simulink model "SimulinkTesting"  (R2019a)
settings: Solver=VariableStepAuto  StartTime=0.0  StopTime=1  MaxStep=0.2  MinStep=0.1  RelTol=1e-3
settings Model: Creator=Devin  LastModifiedBy=Devin

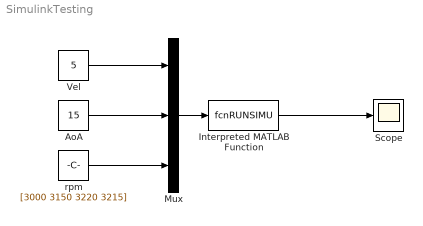
== system SimulinkTesting ==
  AoA : Constant  Value=15
  Interpreted MATLAB Function : MATLABFcn  MATLABFcn=fcnRUNSIMU
  Mux : Mux  Inputs=3
  Scope : Scope
  "Vel " : Constant  Value=5
  "rpm " : Constant  Value=[3000 3150 3220 3215]
  wires:
  "Vel "/1 -> Mux/1
  Mux/1 -> Interpreted MATLAB Function/1
  "rpm "/1 -> Mux/3
  AoA/1 -> Mux/2
  Interpreted MATLAB Function/1 -> Scope/1
